simulink model "p4_sim"  (R2024b)
settings: Solver=VariableStepAuto  StartTime=0.0  StopTime=100.0  RelTol=1e-3
libraries: fuzblock x2
settings Model: Creator=ruben  LastModifiedBy=ruben

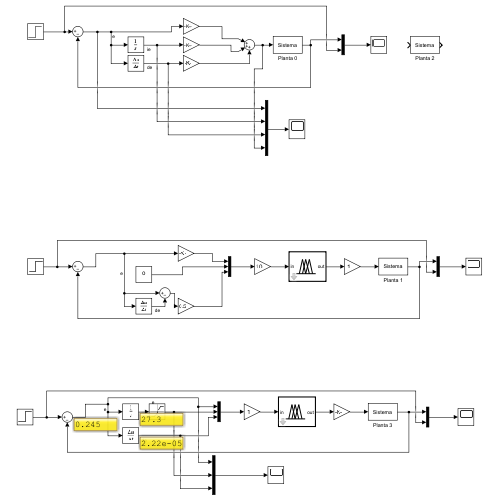
[thumbnail: Simulink's stored preview of the top-level diagram]
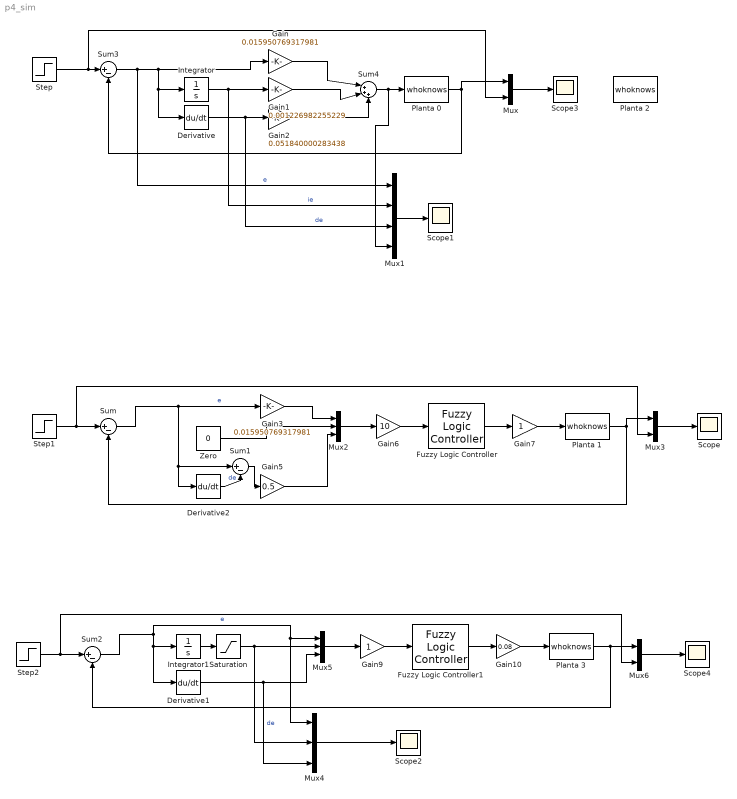
== system p4_sim ==
  Derivative : Derivative
  Derivative1 : Derivative  CoefficientInTFapproximation=0.1
  Derivative2 : Derivative  CoefficientInTFapproximation=0.1
  Fuzzy Logic Controller : fuzblock/Fuzzy Logic  Controller  FIS='pid_fuzzy_2'  OutputSampleNumber=101  DataType=double  FuzzifiedInputs=off  RuleFiringStrengths=off  RuleOutputs=off  AggregatedOutputs=off  SimulateUsing=Interpreted execution  OutOfRangeInputValueMessage=warning  NoRuleFiredMessage=warning  EmptyOutputFuzzySetMessage=warning
  Fuzzy Logic Controller1 : fuzblock/Fuzzy Logic  Controller  FIS='pid_fuzzy_4'  OutputSampleNumber=101  DataType=double  FuzzifiedInputs=off  RuleFiringStrengths=off  RuleOutputs=off  AggregatedOutputs=off  SimulateUsing=Interpreted execution  OutOfRangeInputValueMessage=warning  NoRuleFiredMessage=warning  EmptyOutputFuzzySetMessage=warning
  Gain : Gain  Gain=0.015950769317981
  Gain1 : Gain  Gain=0.001226982255229
  Gain10 : Gain  Gain=0.08
  Gain2 : Gain  Gain=0.051840000283438
  Gain3 : Gain  Gain=0.015950769317981
  Gain5 : Gain  Gain=0.5
  Gain6 : Gain  Gain=10
  Gain7 : Gain
  Gain9 : Gain
  Integrator : Integrator
  Integrator1 : Integrator
  Mux : Mux  Inputs=2
  Mux1 : Mux
  Mux2 : Mux  Inputs=3
  Mux3 : Mux  Inputs=2
  Mux4 : Mux  Inputs=3
  Mux5 : Mux  Inputs=3
  Mux6 : Mux  Inputs=2
  Planta 0 : M-S-Function  FunctionName=whoknows  Parameters=L, P1, P2, T, R  mask{L=6, P1=2, P2=0, T=1, R=0}
      mask prompts: L "Laboratorio"; P1 "Primer digito del Puesto"; P2 "Segundo digito del Puesto"; T "Tipo de Planta"; R "Ruido"
      mask Display: disp('Sistema')
  Planta 1 : M-S-Function  FunctionName=whoknows  Parameters=L, P1, P2, T, R  mask{L=6, P1=2, P2=0, T=1, R=0}
      mask prompts: L "Laboratorio"; P1 "Primer digito del Puesto"; P2 "Segundo digito del Puesto"; T "Tipo de Planta"; R "Ruido"
      mask Display: disp('Sistema')
  Planta 2 : M-S-Function  FunctionName=whoknows  Parameters=L, P1, P2, T, R  mask{L=6, P1=2, P2=0, T=1, R=0}
      mask prompts: L "Laboratorio"; P1 "Primer digito del Puesto"; P2 "Segundo digito del Puesto"; T "Tipo de Planta"; R "Ruido"
      mask Display: disp('Sistema')
  Planta 3 : M-S-Function  FunctionName=whoknows  Parameters=L, P1, P2, T, R  mask{L=6, P1=2, P2=0, T=1, R=0}
      mask prompts: L "Laboratorio"; P1 "Primer digito del Puesto"; P2 "Segundo digito del Puesto"; T "Tipo de Planta"; R "Ruido"
      mask Display: disp('Sistema')
  Saturation : Saturate  UpperLimit=10  LowerLimit=-10
  Scope{,1..4} (5 alike) : Scope
  Step : Step  Time=0  SampleTime=0
  Step1 : Step  Time=0  SampleTime=0
  Step2 : Step  Time=0  SampleTime=0
  Sum{,1..3} (4 alike) : Sum  Inputs=|+-
  Sum4 : Sum  Inputs=|+++
  Zero : Constant  Value=0  OutDataTypeStr=Inherit: Inherit via back propagation
  wires:
  Sum3/1 -> Mux1/1, Integrator/1, Derivative/1, Gain/1  "e"
  Sum4/1 -> Mux1/4, Planta 0/1
  Planta 0/1 -> Mux/1, Sum3/2
  Gain2/1 -> Sum4/3
  Step/1 -> Mux/2, Sum3/1
  Derivative/1 -> Mux1/3, Gain2/1  "de"
  Integrator/1 -> Mux1/2, Gain1/1  "ie"
  Gain1/1 -> Sum4/2
  Gain/1 -> Sum4/1
  Step1/1 -> Mux3/2, Sum/1
  Mux/1 -> Scope3/1
  Mux1/1 -> Scope1/1
  Planta 1/1 -> Sum/2, Mux3/1
  Sum/1 -> Derivative2/1, Sum1/1, Gain3/1  "e"
  Derivative2/1 -> Sum1/2  "de"
  Gain3/1 -> Mux2/1
  Mux2/1 -> Gain6/1
  Fuzzy Logic Controller/1 -> Gain7/1
  Gain6/1 -> Fuzzy Logic Controller/1
  Gain7/1 -> Planta 1/1
  Gain5/1 -> Mux2/3
  Sum1/1 -> Gain5/1
  Mux3/1 -> Scope/1
  Zero/1 -> Mux2/2
  Gain10/1 -> Planta 3/1
  Planta 3/1 -> Sum2/2, Mux6/1
  Mux5/1 -> Gain9/1
  Gain9/1 -> Fuzzy Logic Controller1/1
  Step2/1 -> Mux6/2, Sum2/1
  Sum2/1 -> Mux4/1, Mux5/1, Integrator1/1, Derivative1/1  "e"
  Fuzzy Logic Controller1/1 -> Gain10/1
  Mux6/1 -> Scope4/1
  Mux4/1 -> Scope2/1
  Derivative1/1 -> Mux4/3, Mux5/3  "de"
  Integrator1/1 -> Saturation/1
  Saturation/1 -> Mux4/2, Mux5/2
